simulink model "half_band"  (Simulink 7.4)
settings: Solver=ode45  StartTime=0.0  StopTime=10.0  RelTol=1e-3
libraries: xbsIndex_r4 x300, casper_library_downconverter x96, casper_library_misc x24
(part 6 of 6)

== system half_band/parallel_fir4/f0pf1/fir_col7 ==
  real1 : Inport
  imag1 : Inport  Port=2
  fir_tap1 : casper_library_downconverter/fir_tap  SystemSampleTime=-1  factor=0.7  latency=2  coeff_bit_width=25  coeff_bin_pt=24
  real_out1 : Outport
  imag_out1 : Outport  Port=2
  real_sum : Outport  Port=3
  imag_sum : Outport  Port=4
  wires:
  fir_tap1/4 -> imag_sum/1
  fir_tap1/3 -> real_sum/1
  fir_tap1/2 -> imag_out1/1
  fir_tap1/1 -> real_out1/1
  imag1/1 -> fir_tap1/2
  real1/1 -> fir_tap1/1

== system half_band/parallel_fir4/f0pf1/fir_col8 ==
  real1 : Inport
  imag1 : Inport  Port=2
  fir_tap1 : casper_library_downconverter/fir_tap  SystemSampleTime=-1  factor=0.8  latency=2  coeff_bit_width=25  coeff_bin_pt=24
  real_out1 : Outport
  imag_out1 : Outport  Port=2
  real_sum : Outport  Port=3
  imag_sum : Outport  Port=4
  wires:
  fir_tap1/4 -> imag_sum/1
  fir_tap1/3 -> real_sum/1
  fir_tap1/2 -> imag_out1/1
  fir_tap1/1 -> real_out1/1
  imag1/1 -> fir_tap1/2
  real1/1 -> fir_tap1/1

== system half_band/parallel_fir4/f0pf1/imag_sum ==
  sync : Inport
  din1 : Inport  Port=2
  din2 : Inport  Port=3
  din3 : Inport  Port=4
  din4 : Inport  Port=5
  din5 : Inport  Port=6
  din6 : Inport  Port=7
  din7 : Inport  Port=8
  din8 : Inport  Port=9
  addr{1..7} (7 alike) : xbsIndex_r4/AddSub  mode=Addition  use_carryin=off  use_carryout=off  en=off  latency=1  precision=Full  arith_type=Unsigned  n_bits=16  bin_pt=14  quantization=Truncate  overflow=Wrap  dbl_ovrd=off  use_behavioral_HDL=off  hw_selection=Fabric  pipelined=on  use_rpm=on  block_type=addsub
      addr1 settings: block_version=10.1.3
      addr2 settings: block_version=10.1.3
      addr3 settings: block_version=10.1.3
  sync_delay : xbsIndex_r4/Delay  en=off  latency=3  dbl_ovrd=off  reg_retiming=on  block_type=delay
  sync_out : Outport
  dout : Outport  Port=2
  wires:
  addr7/1 -> dout/1
  addr6/1 -> addr7/2
  addr5/1 -> addr7/1
  addr4/1 -> addr6/2
  addr3/1 -> addr6/1
  addr2/1 -> addr5/2
  addr1/1 -> addr5/1
  din8/1 -> addr4/2
  din7/1 -> addr4/1
  din6/1 -> addr3/2
  din5/1 -> addr3/1
  din4/1 -> addr2/2
  din3/1 -> addr2/1
  din2/1 -> addr1/2
  din1/1 -> addr1/1
  sync_delay/1 -> sync_out/1
  sync/1 -> sync_delay/1

== system half_band/parallel_fir4/f0pf1/real_sum ==
  sync : Inport
  din1 : Inport  Port=2
  din2 : Inport  Port=3
  din3 : Inport  Port=4
  din4 : Inport  Port=5
  din5 : Inport  Port=6
  din6 : Inport  Port=7
  din7 : Inport  Port=8
  din8 : Inport  Port=9
  addr{1..7} (7 alike) : xbsIndex_r4/AddSub  mode=Addition  use_carryin=off  use_carryout=off  en=off  latency=1  precision=Full  arith_type=Unsigned  n_bits=16  bin_pt=14  quantization=Truncate  overflow=Wrap  dbl_ovrd=off  use_behavioral_HDL=off  hw_selection=Fabric  pipelined=on  use_rpm=on  block_type=addsub
      addr1 settings: block_version=10.1.3
      addr2 settings: block_version=10.1.3
      addr3 settings: block_version=10.1.3
  sync_delay : xbsIndex_r4/Delay  en=off  latency=3  dbl_ovrd=off  reg_retiming=on  block_type=delay
  sync_out : Outport
  dout : Outport  Port=2
  wires:
  addr7/1 -> dout/1
  addr6/1 -> addr7/2
  addr5/1 -> addr7/1
  addr4/1 -> addr6/2
  addr3/1 -> addr6/1
  addr2/1 -> addr5/2
  addr1/1 -> addr5/1
  din8/1 -> addr4/2
  din7/1 -> addr4/1
  din6/1 -> addr3/2
  din5/1 -> addr3/1
  din4/1 -> addr2/2
  din3/1 -> addr2/1
  din2/1 -> addr1/2
  din1/1 -> addr1/1
  sync_delay/1 -> sync_out/1
  sync/1 -> sync_delay/1

== system half_band/parallel_fir4/f1/fir_col1 ==
  real1 : Inport
  imag1 : Inport  Port=2
  fir_tap1 : casper_library_downconverter/fir_tap  SystemSampleTime=-1  factor=0.1  latency=2  coeff_bit_width=25  coeff_bin_pt=24
  real_out1 : Outport
  imag_out1 : Outport  Port=2
  real_sum : Outport  Port=3
  imag_sum : Outport  Port=4
  wires:
  real1/1 -> fir_tap1/1
  imag1/1 -> fir_tap1/2
  fir_tap1/1 -> real_out1/1
  fir_tap1/2 -> imag_out1/1
  fir_tap1/3 -> real_sum/1
  fir_tap1/4 -> imag_sum/1

== system half_band/parallel_fir4/f1/fir_col2 ==
  real1 : Inport
  imag1 : Inport  Port=2
  fir_tap1 : casper_library_downconverter/fir_tap  SystemSampleTime=-1  factor=0.2  latency=2  coeff_bit_width=25  coeff_bin_pt=24
  real_out1 : Outport
  imag_out1 : Outport  Port=2
  real_sum : Outport  Port=3
  imag_sum : Outport  Port=4
  wires:
  real1/1 -> fir_tap1/1
  imag1/1 -> fir_tap1/2
  fir_tap1/1 -> real_out1/1
  fir_tap1/2 -> imag_out1/1
  fir_tap1/3 -> real_sum/1
  fir_tap1/4 -> imag_sum/1

== system half_band/parallel_fir4/f1/fir_col3 ==
  real1 : Inport
  imag1 : Inport  Port=2
  fir_tap1 : casper_library_downconverter/fir_tap  SystemSampleTime=-1  factor=0.3  latency=2  coeff_bit_width=25  coeff_bin_pt=24
  real_out1 : Outport
  imag_out1 : Outport  Port=2
  real_sum : Outport  Port=3
  imag_sum : Outport  Port=4
  wires:
  real1/1 -> fir_tap1/1
  imag1/1 -> fir_tap1/2
  fir_tap1/1 -> real_out1/1
  fir_tap1/2 -> imag_out1/1
  fir_tap1/3 -> real_sum/1
  fir_tap1/4 -> imag_sum/1

== system half_band/parallel_fir4/f1/fir_col4 ==
  real1 : Inport
  imag1 : Inport  Port=2
  fir_tap1 : casper_library_downconverter/fir_tap  SystemSampleTime=-1  factor=0.4  latency=2  coeff_bit_width=25  coeff_bin_pt=24
  real_out1 : Outport
  imag_out1 : Outport  Port=2
  real_sum : Outport  Port=3
  imag_sum : Outport  Port=4
  wires:
  real1/1 -> fir_tap1/1
  imag1/1 -> fir_tap1/2
  fir_tap1/1 -> real_out1/1
  fir_tap1/2 -> imag_out1/1
  fir_tap1/3 -> real_sum/1
  fir_tap1/4 -> imag_sum/1

== system half_band/parallel_fir4/f1/fir_col5 ==
  real1 : Inport
  imag1 : Inport  Port=2
  fir_tap1 : casper_library_downconverter/fir_tap  SystemSampleTime=-1  factor=0.5  latency=2  coeff_bit_width=25  coeff_bin_pt=24
  real_out1 : Outport
  imag_out1 : Outport  Port=2
  real_sum : Outport  Port=3
  imag_sum : Outport  Port=4
  wires:
  real1/1 -> fir_tap1/1
  imag1/1 -> fir_tap1/2
  fir_tap1/1 -> real_out1/1
  fir_tap1/2 -> imag_out1/1
  fir_tap1/3 -> real_sum/1
  fir_tap1/4 -> imag_sum/1

== system half_band/parallel_fir4/f1/fir_col6 ==
  real1 : Inport
  imag1 : Inport  Port=2
  fir_tap1 : casper_library_downconverter/fir_tap  SystemSampleTime=-1  factor=0.6  latency=2  coeff_bit_width=25  coeff_bin_pt=24
  real_out1 : Outport
  imag_out1 : Outport  Port=2
  real_sum : Outport  Port=3
  imag_sum : Outport  Port=4
  wires:
  real1/1 -> fir_tap1/1
  imag1/1 -> fir_tap1/2
  fir_tap1/1 -> real_out1/1
  fir_tap1/2 -> imag_out1/1
  fir_tap1/3 -> real_sum/1
  fir_tap1/4 -> imag_sum/1

== system half_band/parallel_fir4/f1/fir_col7 ==
  real1 : Inport
  imag1 : Inport  Port=2
  fir_tap1 : casper_library_downconverter/fir_tap  SystemSampleTime=-1  factor=0.7  latency=2  coeff_bit_width=25  coeff_bin_pt=24
  real_out1 : Outport
  imag_out1 : Outport  Port=2
  real_sum : Outport  Port=3
  imag_sum : Outport  Port=4
  wires:
  real1/1 -> fir_tap1/1
  imag1/1 -> fir_tap1/2
  fir_tap1/1 -> real_out1/1
  fir_tap1/2 -> imag_out1/1
  fir_tap1/3 -> real_sum/1
  fir_tap1/4 -> imag_sum/1

== system half_band/parallel_fir4/f1/fir_col8 ==
  real1 : Inport
  imag1 : Inport  Port=2
  fir_tap1 : casper_library_downconverter/fir_tap  SystemSampleTime=-1  factor=0.8  latency=2  coeff_bit_width=25  coeff_bin_pt=24
  real_out1 : Outport
  imag_out1 : Outport  Port=2
  real_sum : Outport  Port=3
  imag_sum : Outport  Port=4
  wires:
  real1/1 -> fir_tap1/1
  imag1/1 -> fir_tap1/2
  fir_tap1/1 -> real_out1/1
  fir_tap1/2 -> imag_out1/1
  fir_tap1/3 -> real_sum/1
  fir_tap1/4 -> imag_sum/1

== system half_band/parallel_fir4/f1/imag_sum ==
  sync : Inport
  din1 : Inport  Port=2
  din2 : Inport  Port=3
  din3 : Inport  Port=4
  din4 : Inport  Port=5
  din5 : Inport  Port=6
  din6 : Inport  Port=7
  din7 : Inport  Port=8
  din8 : Inport  Port=9
  addr{1..7} (7 alike) : xbsIndex_r4/AddSub  mode=Addition  use_carryin=off  use_carryout=off  en=off  latency=1  precision=Full  arith_type=Unsigned  n_bits=16  bin_pt=14  quantization=Truncate  overflow=Wrap  dbl_ovrd=off  use_behavioral_HDL=off  hw_selection=Fabric  pipelined=on  use_rpm=on  block_type=addsub
      addr1 settings: block_version=10.1.3
      addr2 settings: block_version=10.1.3
      addr3 settings: block_version=10.1.3
  sync_delay : xbsIndex_r4/Delay  en=off  latency=3  dbl_ovrd=off  reg_retiming=on  block_type=delay
  sync_out : Outport
  dout : Outport  Port=2
  wires:
  sync/1 -> sync_delay/1
  sync_delay/1 -> sync_out/1
  din1/1 -> addr1/1
  din2/1 -> addr1/2
  din3/1 -> addr2/1
  din4/1 -> addr2/2
  din5/1 -> addr3/1
  din6/1 -> addr3/2
  din7/1 -> addr4/1
  din8/1 -> addr4/2
  addr1/1 -> addr5/1
  addr2/1 -> addr5/2
  addr3/1 -> addr6/1
  addr4/1 -> addr6/2
  addr5/1 -> addr7/1
  addr6/1 -> addr7/2
  addr7/1 -> dout/1

== system half_band/parallel_fir4/f1/real_sum ==
  sync : Inport
  din1 : Inport  Port=2
  din2 : Inport  Port=3
  din3 : Inport  Port=4
  din4 : Inport  Port=5
  din5 : Inport  Port=6
  din6 : Inport  Port=7
  din7 : Inport  Port=8
  din8 : Inport  Port=9
  addr{1..7} (7 alike) : xbsIndex_r4/AddSub  mode=Addition  use_carryin=off  use_carryout=off  en=off  latency=1  precision=Full  arith_type=Unsigned  n_bits=16  bin_pt=14  quantization=Truncate  overflow=Wrap  dbl_ovrd=off  use_behavioral_HDL=off  hw_selection=Fabric  pipelined=on  use_rpm=on  block_type=addsub
      addr1 settings: block_version=10.1.3
      addr2 settings: block_version=10.1.3
      addr3 settings: block_version=10.1.3
  sync_delay : xbsIndex_r4/Delay  en=off  latency=3  dbl_ovrd=off  reg_retiming=on  block_type=delay
  sync_out : Outport
  dout : Outport  Port=2
  wires:
  sync/1 -> sync_delay/1
  sync_delay/1 -> sync_out/1
  din1/1 -> addr1/1
  din2/1 -> addr1/2
  din3/1 -> addr2/1
  din4/1 -> addr2/2
  din5/1 -> addr3/1
  din6/1 -> addr3/2
  din7/1 -> addr4/1
  din8/1 -> addr4/2
  addr1/1 -> addr5/1
  addr2/1 -> addr5/2
  addr3/1 -> addr6/1
  addr4/1 -> addr6/2
  addr5/1 -> addr7/1
  addr6/1 -> addr7/2
  addr7/1 -> dout/1
